simulink model "hvac_nnpid"  (R2026a)
settings: Solver=ode45  StopTime=T_end  MaxStep=10  RelTol=1e-4
PreLoadFcn:
  | init_workspace;
undefined symbols (not defined in the file or in its folder): c_vent, Ca, ctrl_mode, Cw, K_fixed, Ro, Rw, Rwin, sig_Ti, sig_To, tau_act, tau_s, Ti0, To_ts, Ts, Tw0
libraries: sl_discontinuities x1
settings Model: Creator=munna  LastModifiedBy=munna

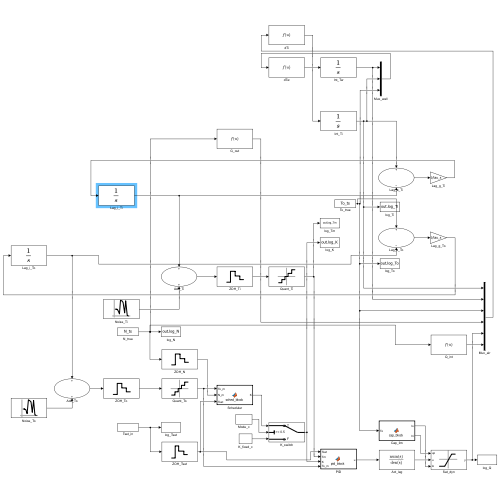
[thumbnail: Simulink's stored preview of the top-level diagram]
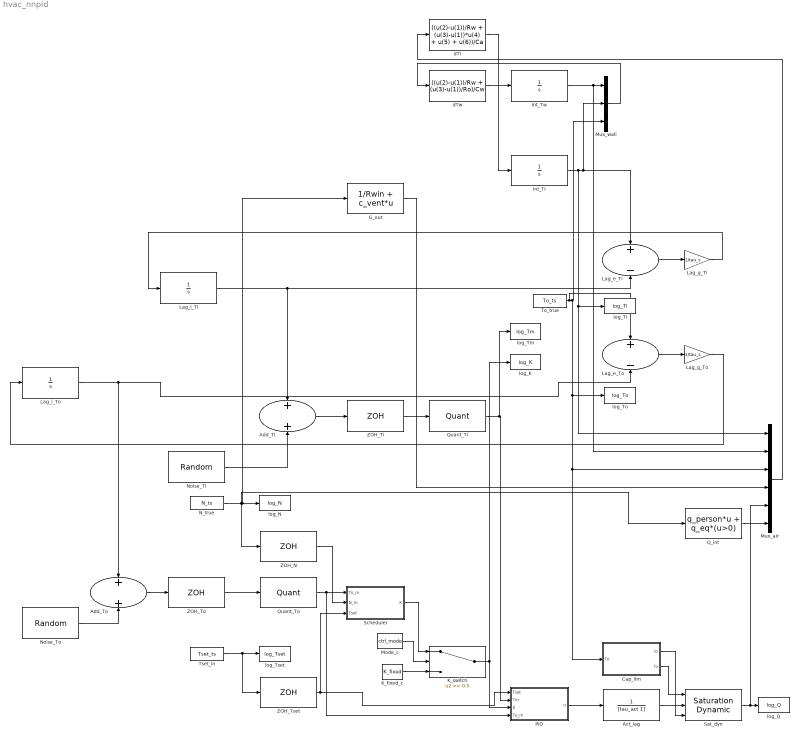
== system hvac_nnpid ==
  Act_lag : TransferFcn  Denominator=[tau_act 1]
  Add_Ti : Sum
  Add_To : Sum
  Cap_lim : MATLAB Function  TreatAsAtomicUnit=on
  G_out : Fcn  Expr=1/Rwin + c_vent*u
  Int_Ti : Integrator  InitialCondition=Ti0
  Int_Tw : Integrator  InitialCondition=Tw0
  K_fixed_c : Constant  Value=K_fixed  VectorParams1D=off
  K_switch : Switch  Threshold=0.5  SaturateOnIntegerOverflow=off  InputSameDT=off
  Lag_e_Ti : Sum  Inputs=+-
  Lag_e_To : Sum  Inputs=+-
  Lag_g_Ti : Gain  Gain=1/tau_s
  Lag_g_To : Gain  Gain=1/tau_s
  Lag_i_Ti : Integrator  InitialCondition=Ti0
  Lag_i_To : Integrator  InitialCondition=To_ts.Data(1)
  Mode_c : Constant  Value=ctrl_mode
  Mux_air : Mux  Inputs=6
  Mux_wall : Mux  Inputs=3
  N_true : FromWorkspace  VariableName=N_ts  Interpolate=off  OutputAfterFinalValue=Holding final value
  Noise_Ti : RandomNumber  Variance=sig_Ti^2  Seed=11  SampleTime=Ts
  Noise_To : RandomNumber  Variance=sig_To^2  Seed=22  SampleTime=Ts
  PID : MATLAB Function  TreatAsAtomicUnit=on
  Q_int : Fcn  Expr=q_person*u + q_eq*(u>0)
  Quant_Ti : Quantizer  QuantizationInterval=q_res
  Quant_To : Quantizer  QuantizationInterval=q_res
  Sat_dyn : sl_discontinuities/Saturation Dynamic  OutMin=[]  OutMax=[]  OutDataTypeStr=Inherit: Same as second input  OutDataType=fixdt(1, 16)  OutScaling=2^-10  DoSatur=off
      settings: LibrarySourceBlock=|
      | simulink/Discontinuities/Saturation
      | Dynamic
  Scheduler : MATLAB Function  TreatAsAtomicUnit=on
  To_true : FromWorkspace  VariableName=To_ts  OutputAfterFinalValue=Holding final value
  Tset_in : FromWorkspace  VariableName=Tset_ts  OutputAfterFinalValue=Holding final value
  ZOH_N : ZeroOrderHold  SampleTime=Ts
  ZOH_Ti : ZeroOrderHold  SampleTime=Ts
  ZOH_To : ZeroOrderHold  SampleTime=Ts
  ZOH_Tset : ZeroOrderHold  SampleTime=Ts
  dTi : Fcn  Expr=((u(2)-u(1))/Rw + (u(3)-u(1))*u(4) + u(5) + u(6))/Ca
  dTw : Fcn  Expr=((u(2)-u(1))/Rw + (u(3)-u(1))/Ro)/Cw
  log_K : ToWorkspace  VariableName=log_K  SaveFormat=Timeseries  SampleTime=-1
  log_N : ToWorkspace  VariableName=log_N  SaveFormat=Timeseries  SampleTime=-1
  log_Q : ToWorkspace  VariableName=log_Q  SaveFormat=Timeseries  SampleTime=-1
  log_Ti : ToWorkspace  VariableName=log_Ti  SaveFormat=Timeseries  SampleTime=-1
  log_Tm : ToWorkspace  VariableName=log_Tm  SaveFormat=Timeseries  SampleTime=-1
  log_To : ToWorkspace  VariableName=log_To  SaveFormat=Timeseries  SampleTime=-1
  log_Tset : ToWorkspace  VariableName=log_Tset  SaveFormat=Timeseries  SampleTime=-1
  wires:
  Lag_e_To/1 -> Lag_g_To/1
  Noise_To/1 -> Add_To/2
  Add_To/1 -> ZOH_To/1
  Lag_i_To/1 -> Add_To/1, Lag_e_To/2
  Add_Ti/1 -> ZOH_Ti/1
  Lag_i_Ti/1 -> Add_Ti/1, Lag_e_Ti/2
  Noise_Ti/1 -> Add_Ti/2
  To_true/1 -> Mux_air/3, Cap_lim/1(To), log_To/1, Mux_wall/3, Lag_e_To/1
  N_true/1 -> G_out/1, log_N/1, ZOH_N/1, Q_int/1
  ZOH_To/1 -> Quant_To/1
  Tset_in/1 -> log_Tset/1, ZOH_Tset/1
  ZOH_N/1 -> Scheduler/2(N_m)
  Quant_To/1 -> PID/4(To_m), Scheduler/1(To_m)
  ZOH_Tset/1 -> PID/1(Tset), Scheduler/3(Tset)
  G_out/1 -> Mux_air/4
  ZOH_Ti/1 -> Quant_Ti/1
  K_fixed_c/1 -> K_switch/3
  Scheduler/1(K) -> K_switch/1
  Mode_c/1 -> K_switch/2
  dTi/1 -> Int_Ti/1
  Sat_dyn/1 -> log_Q/1, Mux_air/5
  Mux_wall/1 -> dTw/1
  Int_Ti/1 -> Mux_air/1, log_Ti/1, Lag_e_Ti/1, Mux_wall/2
  dTw/1 -> Int_Tw/1
  Quant_Ti/1 -> log_Tm/1, PID/2(Tm)
  Lag_e_Ti/1 -> Lag_g_Ti/1
  PID/1(u) -> Act_lag/1
  K_switch/1 -> log_K/1, PID/3(K)
  Int_Tw/1 -> Mux_air/2, Mux_wall/1
  Act_lag/1 -> Sat_dyn/2
  Cap_lim/1(lo) -> Sat_dyn/3
  Cap_lim/2(hi) -> Sat_dyn/1
  Lag_g_Ti/1 -> Lag_i_Ti/1
  Lag_g_To/1 -> Lag_i_To/1
  Q_int/1 -> Mux_air/6
  Mux_air/1 -> dTi/1

== matlab function hvac_nnpid/PID ==
  data: Tset input; u output; Tm input; K input; To_m input
function u = pid_block(Tset, Tm, K, To_m)
persistent I Tm_prev
if isempty(I)
    I = 0;
    Tm_prev = Tm;
end
[u, I] = pid_step(Tset, Tm, K, I, Tm_prev, To_m);
Tm_prev = Tm;
end

== matlab function hvac_nnpid/Scheduler ==
  data: To_m input; K output; N_m input; Tset input
function K = sched_block(To_m, N_m, Tset)
persistent st
if isempty(st)
    st = zeros(4,1);
end
[K, st] = gain_scheduler(To_m, N_m, Tset, st);
end

== matlab function hvac_nnpid/Cap_lim ==
  data: To input; lo output; hi output
function [lo, hi] = cap_block(To)
[Qc, Qh, ~] = hvac_capacity(To);
lo = -Qc;
hi = Qh;
end
